simulink model "Model_Hems"  (R2022b)
settings: Solver=FixedStepAuto  StartTime=0.0  StopTime=10.0  RelTol=1e-3
values from neighbouring files (symbols this model uses):
  hems =     [hems.mat]
undefined symbols (not defined in the file or in its folder): magnitude
settings Model: Creator=ramuj  LastModifiedBy=ramuj

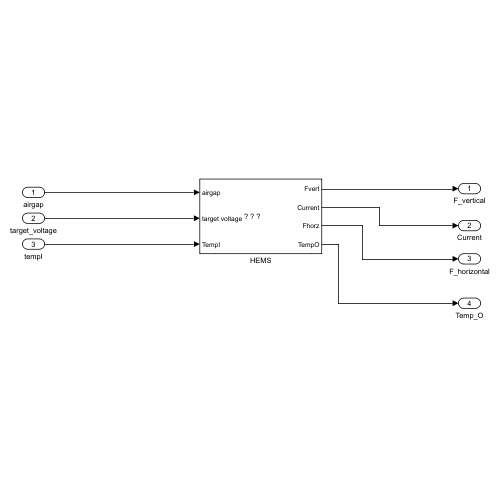
[thumbnail: Simulink's stored preview of the top-level diagram]
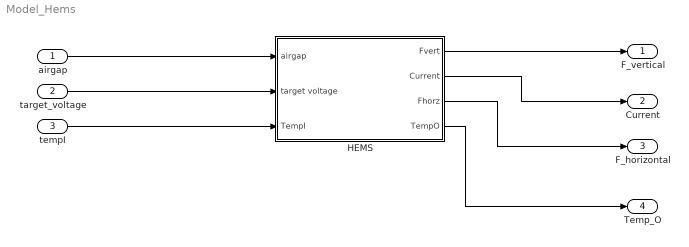
== system Model_Hems ==
  airgap : Inport
  target_voltage : Inport  Port=2
  tempI : Inport  Port=3
  HEMS : Subsystem
      mask Display: image('C:\Users\ramuj\Desktop\Hyperloop\H8\Imagenes o Renders\hems.png'); % Use "Edit Image" on toolstrip to change.
  F_vertical : Outport
  Current : Outport  Port=2
  F_horizontal : Outport  Port=3
  Temp_O : Outport  Port=4
  wires:
  tempI/1 -> HEMS/3(TempI)
  HEMS/1(Fvert) -> F_vertical/1
  HEMS/2(Current) -> Current/1
  HEMS/3(Fhorz) -> F_horizontal/1
  HEMS/4(TempO) -> Temp_O/1
  airgap/1 -> HEMS/1(airgap)
  target_voltage/1 -> HEMS/2(target voltage)

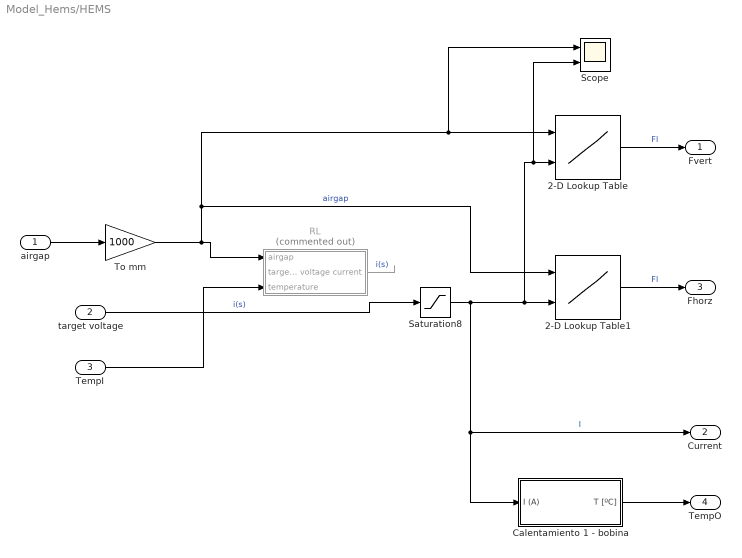
== system Model_Hems/HEMS ==
  airgap : Inport
  target voltage : Inport  Port=2
  TempI : Inport  Port=3
  2-D Lookup Table : Lookup_n-D  BreakpointsForDimension1=hems.Airgap'  BreakpointsForDimension2=hems.Current  Table=hems.Force_Vertical  InternalRulePriority=Speed  RndMeth=Simplest
      settings: InputPortMap=u0,u1
  2-D Lookup Table1 : Lookup_n-D  BreakpointsForDimension1=hems.Airgap'  BreakpointsForDimension2=hems.Current  Table=hems.Force_Horizontal  InternalRulePriority=Speed  RndMeth=Simplest
      settings: InputPortMap=u0,u1
  Calentamiento 1 - bobina : Subsystem
  RL : Subsystem  Commented=on
  Saturation8 : Saturate  UpperLimit=50  LowerLimit=-50
  Scope : Scope  NumInputPorts=2
  To mm : Gain  Gain=1000
  Fvert : Outport
  Current : Outport  Port=2
  Fhorz : Outport  Port=3
  TempO : Outport  Port=4
  wires:
  2-D Lookup Table/1 -> Fvert/1  "Fl"
  airgap/1 -> To mm/1
  Saturation8/1 -> Calentamiento 1 - bobina/1(I (A)), Current/1, 2-D Lookup Table1/2, Scope/2, 2-D Lookup Table/2  "I"
  target voltage/1 -> Saturation8/1  "i(s)"
  TempI/1 -> RL/3(temperature)
  2-D Lookup Table1/1 -> Fhorz/1  "Fl"
  Calentamiento 1 - bobina/1(T [ºC]) -> TempO/1
  To mm/1 -> Scope/1, 2-D Lookup Table/1, 2-D Lookup Table1/1, RL/1(airgap)  "airgap"
  RL/1(current) -> ?  "i(s)"

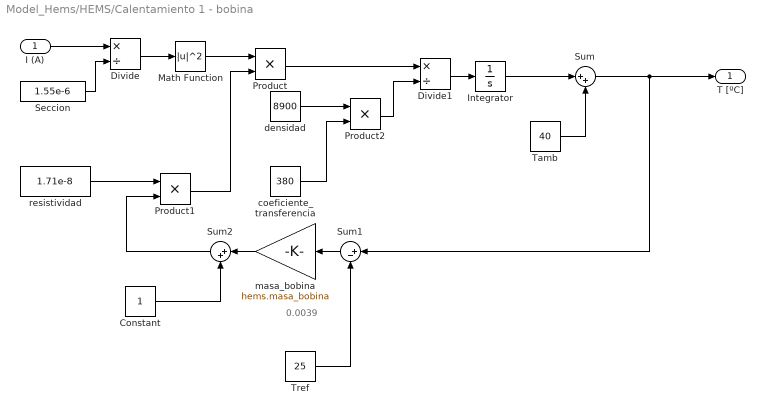
== system Model_Hems/HEMS/Calentamiento 1 - bobina ==
  note: 0.0039
  I (A) : Inport
  Constant : Constant
  Divide : Product  Inputs=*/
  Divide1 : Product  Inputs=*/
  Integrator : Integrator
  Math Function : Math  Operator=magnitude^2
  Product : Product
  Product1 : Product
  Product2 : Product
  Seccion : Constant  Value=1.55e-6
  Sum : Sum  Inputs=|++
  Sum1 : Sum  Inputs=|+-
  Sum2 : Sum  Inputs=|++
  Tamb : Constant  Value=40
  Tref : Constant  Value=25
  coeficiente_transferencia : Constant  Value=380
  densidad : Constant  Value=8900
  masa_bobina : Gain  Gain=hems.masa_bobina
  resistividad : Constant  Value=1.71e-8
  T [ºC] : Outport
  wires:
  I (A)/1 -> Divide/1
  Seccion/1 -> Divide/2
  Divide/1 -> Math Function/1
  Math Function/1 -> Product/1
  Product/1 -> Divide1/1
  Divide1/1 -> Integrator/1
  Integrator/1 -> Sum/1
  Tamb/1 -> Sum/2
  Sum/1 -> Sum1/1, T [ºC]/1
  Sum1/1 -> masa_bobina/1
  Tref/1 -> Sum1/2
  masa_bobina/1 -> Sum2/1
  Constant/1 -> Sum2/2
  resistividad/1 -> Product1/1
  Sum2/1 -> Product1/2
  Product1/1 -> Product/2
  Product2/1 -> Divide1/2
  densidad/1 -> Product2/1
  coeficiente_transferencia/1 -> Product2/2

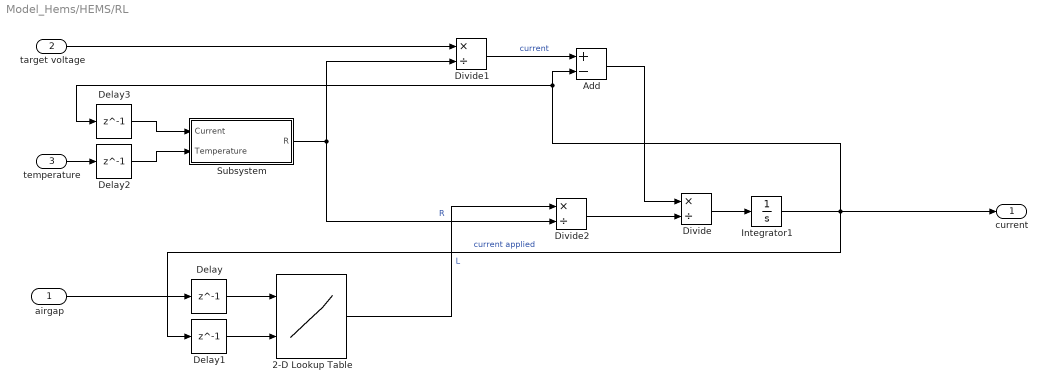
== system Model_Hems/HEMS/RL ==
  airgap : Inport
  target voltage : Inport  Port=2
  temperature : Inport  Port=3
  2-D Lookup Table : Lookup_n-D  BreakpointsForDimension1=hems.Airgap  BreakpointsForDimension2=hems.Current(2:110)  Table=hems.Inductance  InternalRulePriority=Speed  RndMeth=Simplest
      settings: InputPortMap=u0,u1
  Add : Sum  Inputs=+-
  Delay{,1..3} (4 alike) : Delay  DelayLength=1
  Divide : Product  Inputs=*/
  Divide1 : Product  Inputs=*/
  Divide2 : Product  Inputs=*/
  Integrator1 : Integrator
  Subsystem : Subsystem
  current : Outport
  wires:
  airgap/1 -> Delay/1
  Divide/1 -> Integrator1/1
  Add/1 -> Divide/1
  Integrator1/1 -> Delay1/1, current/1, Delay3/1, Add/2  "current applied"
  2-D Lookup Table/1 -> Divide2/1  "L"
  target voltage/1 -> Divide1/1
  temperature/1 -> Delay2/1
  Divide1/1 -> Add/1  "current"
  Subsystem/1(R) -> Divide2/2, Divide1/2  "R"
  Delay3/1 -> Subsystem/1(Current)
  Delay2/1 -> Subsystem/2(Temperature)
  Divide2/1 -> Divide/2
  Delay1/1 -> 2-D Lookup Table/2
  Delay/1 -> 2-D Lookup Table/1

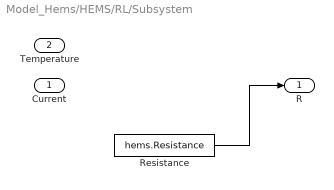
== system Model_Hems/HEMS/RL/Subsystem ==
  Current : Inport
  Temperature : Inport  Port=2
  Resistance : Constant  Value=hems.Resistance
  R : Outport
  wires:
  Resistance/1 -> R/1
